simulink model "fz4_7"  (R2014a)
settings: Solver=ode45  StartTime=0.0  StopTime=10.0  RelTol=1e-3
libraries: commutil2 x4, commsink2 x2, commfilt2 x2, commdigbbndpm3 x2, commchan3 x1, commrandsrc2 x1
settings Model: Creator=tzb  LastModifiedBy=tzb
settings DebuggingCC: SolverPrmCheckMsg=none

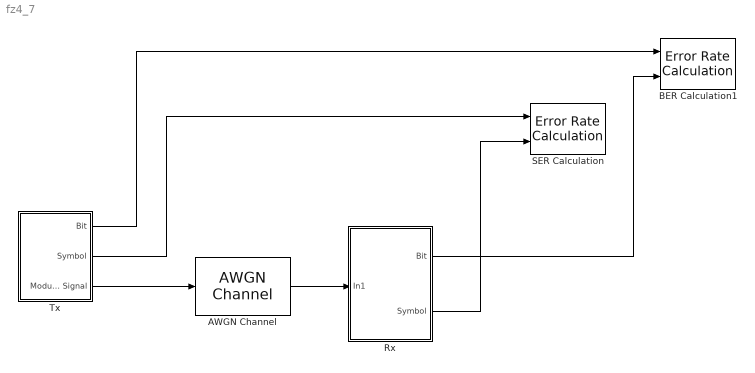
== system fz4_7 ==
  AWGN Channel : commchan3/AWGN Channel  InputProcessing=Columns as channels (frame based)  seed=123456  noiseMode="Signal to noise ratio  (SNR)"  EbNodB=10  EsNodB=10  SNRdB=SNR  bitsPerSym=1  Ps=1  Tsym=1  variance=1
  BER Calculation1 : commsink2/Error Rate Calculation  N=0  st_delay=0  cp_mode=Entire frame  subframe=[]  PMode=Workspace  WsName=BER  RsMode2=off  stop=off  numErr=100  maxBits=1e6
  Rx : Subsystem
  SER Calculation : commsink2/Error Rate Calculation  N=0  st_delay=0  cp_mode=Entire frame  subframe=[]  PMode=Workspace  WsName=SER  RsMode2=off  stop=off  numErr=100  maxBits=1e6
  Tx : Subsystem
  wires:
  Tx/3(Modulated Signal) -> AWGN Channel/1
  AWGN Channel/1 -> Rx/1(In1)
  Tx/1("Bit ") -> BER Calculation1/1
  Tx/2(Symbol) -> SER Calculation/1
  Rx/1(Bit) -> BER Calculation1/2
  Rx/2(Symbol) -> SER Calculation/2

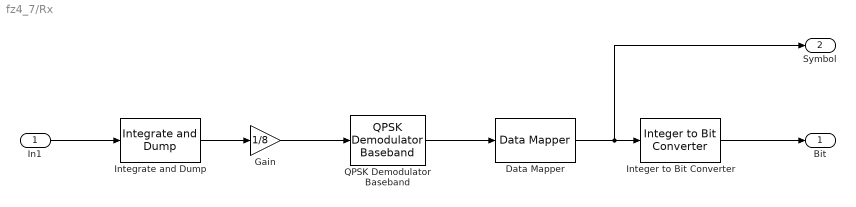
== system fz4_7/Rx ==
  In1 : Inport
  Data Mapper : commutil2/Data Mapper  MapMode=Binary to Gray  M=4  MapVec=[0 1 3 2 7 6 4 5]
  Gain : Gain  Gain=1/8
  Integer to Bit Converter : commutil2/Integer to Bit Converter  nbits=2  signedInputValues=Unsigned  bitOrder=MSB first  outDtype=Inherit via internal rule
  Integrate and Dump : commfilt2/Integrate and Dump  obssamples=8  offsetsamples=0  nodump=off  roundingMode=Floor  overflowMode=off
  QPSK Demodulator Baseband : commdigbbndpm3/QPSK Demodulator Baseband  Ph=0  Dec=Gray  OutType=Integer  DecType=Hard decision  VarSource=Dialog  Variance=1  outDtype1=Inherit via internal rule  outDtype2=Inherit via internal rule  derotateFactorWordLen=16
  Bit : Outport
  Symbol : Outport  Port=2
  wires:
  Integrate and Dump/1 -> Gain/1
  QPSK Demodulator Baseband/1 -> Data Mapper/1
  Data Mapper/1 -> Symbol/1, Integer to Bit Converter/1
  In1/1 -> Integrate and Dump/1
  Gain/1 -> QPSK Demodulator Baseband/1
  Integer to Bit Converter/1 -> Bit/1

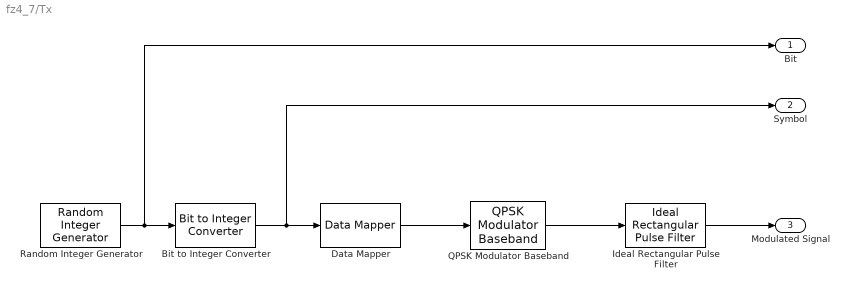
== system fz4_7/Tx ==
  Bit to Integer Converter : commutil2/Bit to Integer Converter  nbits=2  bitOrder=MSB first  signedOutputValues=Unsigned  outDtype=Inherit via internal rule  outDtypeSigned=Inherit via internal rule
  Data Mapper : commutil2/Data Mapper  MapMode=Binary to Gray  M=4  MapVec=[0 1 3 2 7 6 4 5]
  Ideal Rectangular Pulse Filter : commfilt2/Ideal Rectangular Pulse Filter  pulseLen=8  pulseDelay=0  sampMode=Enforce single-rate processing  InputProcessing=Columns as channels (frame based)  normCheck=off  normMode=Sum of samples  filterGain=1  roundingMode=Floor  overflowMode=off
  QPSK Modulator Baseband : commdigbbndpm3/QPSK Modulator Baseband  InType=Integer  Enc=Gray  Ph=0  outDtype=double  outWordLen=16  outUDDataType=sfix(16)  outFracLenMode=Best precision  outFracLen=15
  Random Integer Generator : commrandsrc2/Random Integer Generator  mul=2  seed=37  Ts=1/400000  frameBased=on  sampPerFrame=400000  orient=off  outDataType=double
  "Bit " : Outport
  Symbol : Outport  Port=2
  Modulated Signal : Outport  Port=3
  wires:
  Data Mapper/1 -> QPSK Modulator Baseband/1
  Bit to Integer Converter/1 -> Symbol/1, Data Mapper/1
  QPSK Modulator Baseband/1 -> Ideal Rectangular Pulse Filter/1
  Random Integer Generator/1 -> "Bit "/1, Bit to Integer Converter/1
  Ideal Rectangular Pulse Filter/1 -> Modulated Signal/1
